simulink model "BaseEngineController_LS"  (Simulink 7.7)
settings: Solver=FixedStepDiscrete  StartTime=0.0  StopTime=10.0  RelTol=1e-3
PreLoadFcn:
  | try, eval([bdroot '_setup']); catch, eval('model_setup', ''); end
InitFcn:
  | try, eval([bdroot '_setup']); catch, eval('model_setup', ''); end
undefined symbols (not defined in the file): ECU555, High, motohawk_build_version, motohawk_trunc_name, motohawk_vardec_config_group, motohawk_vardec_path, True
libraries: MotoHawk_lib x1418, motohawk_control_primitives_lib x183, motohawk_engine_lib x32, simulink x21, motohawk_annotations_lib x9, AutoDoc_lib x8, simulink_extras x4, motohawk_ccp_examples_lib x1, motohawk_control_primitives_motoshare_lib x1
(part 11 of 27)

== system BaseEngineController_LS/Foreground/Control/ActuatorCharacterization/Electronic Throttle Controller/ETC Sticking Fault ==
  ETC Error : Inport
  ETC Setpoint Mode : Inport  Port=2
  Abs : Abs
  Logical Operator : Logic  AllPortsSameDT=off  OutDataTypeStr=boolean
  Relational Operator4 : RelationalOperator  Operator=>  ZeroCross=off  InputSameDT=on
  ShutDownAdaptMode1 : motohawk_control_primitives_lib/CompareTo  SystemSampleTime=-1  op===  val=0
  motohawk_calibration1 : MotoHawk_lib/Calibration & Probing Blocks/motohawk_calibration  nam='ETC_StickingThresh'  val=20  storage=Calibration  show_more=on  name_source=Use Parameter  data_type=double  read_level=1  write_level=1  ovr_cals=on  view_as=Number  enum_struct={'Disabled', 'Enabled'}  vector_style=Wide Row  use_help_units=on  help='Defines error limit between TPS_Request and TPS where ETC sticking fault will be set.'  units='%'  use_header_enum=off  row_header_enum={}  col_header_enum={}  use_min_max=on  min_val=-inf  max_val=inf  use_precision=off  precision=''  gain=1  offset=0  exp=1  use_mototune_group=on  mototune_group=motohawk_vardec_path(gcb)
  motohawk_fault_def1 : MotoHawk_lib/Fault Management Blocks/motohawk_fault_def  nam='ETC_Sticking'  mode=Sticky  id=[]  x=254  y=255  input_suspected=on  indeterminate=off  increment_xy=on  downsample_count=1  ovr_cals=on  ovr_actions=on  show_actions=off  action1_name=''  action1_cond=(None)  action2_name=''  action2_cond=(None)  action3_name=''  action3_cond=(None)  action4_name=''  action4_cond=(None)
  wires:
  Abs/1 -> Relational Operator4/1
  motohawk_calibration1/1 -> Relational Operator4/2
  ETC Error/1 -> Abs/1
  Logical Operator/1 -> motohawk_fault_def1/1
  Relational Operator4/1 -> Logical Operator/1
  ShutDownAdaptMode1/1 -> Logical Operator/2
  ETC Setpoint Mode/1 -> ShutDownAdaptMode1/1

== system BaseEngineController_LS/Foreground/Control/ActuatorCharacterization/Electronic Throttle Controller/ETCStallShutDown ==
  Constant1 : Constant  Value=150  OutDataTypeStr=Inherit: Inherit via back propagation  SampleTime=-1
  Logical Operator : Logic  AllPortsSameDT=off  OutDataTypeStr=boolean
  Relational Operator : RelationalOperator  Operator=>  ZeroCross=off  InputSameDT=on
  Relational Operator6 : RelationalOperator  Operator=>  OutDataTypeStr=boolean
  motohawk_ain_read : MotoHawk_lib/Analog I//O Blocks/motohawk_ain_read  nam='ECUP'  typ=uint16
  motohawk_calibration4 : MotoHawk_lib/Calibration & Probing Blocks/motohawk_calibration  nam='ETCShutdownTimerThresh'  val=5  storage=Calibration  show_more=on  name_source=Use Parameter  data_type=double  read_level=1  write_level=1  ovr_cals=on  view_as=Number  enum_struct={'Disabled', 'Enabled'}  vector_style=Wide Row  use_help_units=on  help='Time limit in Stall State after which ETC will shutdown.'  units='s'  use_header_enum=off  row_header_enum={}  col_header_enum={}  use_min_max=on  min_val=-inf  max_val=inf  use_precision=off  precision=''  gain=1  offset=0  exp=1  use_mototune_group=on  mototune_group=motohawk_vardec_path(gcb)
  motohawk_data_read : MotoHawk_lib/Data Storage Blocks/motohawk_data_read  source=Lookup By Name  structure=Scalar  operation=Read scalar from location by index  sz_vec=4  sz_row=2  sz_col=3  typ=double  nam='TimeSinceStall'  checkNull=on  struct_inst_name='Struct1'  struct_nam='MyStruct'
  motohawk_probe : MotoHawk_lib/Calibration & Probing Blocks/motohawk_probe  nam='ETCStallStateShutdown'  show_more=on  name_source=Use Parameter  read_level=1  view_as=Enumeration  enum_struct={'Disabled', 'Enabled'}  vector_style=Wide Row  use_help_units=off  help=''  units=''  use_header_enum=off  row_header_enum={}  col_header_enum={}  use_precision=off  precision=''  gain=1  offset=0  exp=1  use_mototune_group=on  mototune_group=motohawk_vardec_path(gcb)
  State : Outport
  wires:
  motohawk_data_read/1 -> Relational Operator6/1
  motohawk_calibration4/1 -> Relational Operator6/2
  motohawk_ain_read/1 -> Relational Operator/1
  Constant1/1 -> Relational Operator/2
  Relational Operator6/1 -> Logical Operator/1
  Relational Operator/1 -> Logical Operator/2
  Logical Operator/1 -> State/1, motohawk_probe/1

== system BaseEngineController_LS/Foreground/Control/ActuatorCharacterization/Electronic Throttle Controller/PID With Damper Terms (Tunable) ==
  Actual : Inport
  SetPoint : Inport  Port=2
  ResetITerm : Inport  Port=3
  Add : Sum  Inputs=+-
  DamperSwitch : Subsystem
  Ground2 : Ground
  IGain : Subsystem
  PGain : Subsystem
  PID With Damper Terms : Subsystem  Description=|  AncestorBlock=motohawk_control_primitives_lib/PID With Damper Terms  mask(PID with Damper Terms){samp_time=-1}
      | /* Name: ErrorGain Unit:mult ClassID:VAR StorageID:FLASH Access:RW4+RW3+NA2+NA1 TypeID:UINT4                   
      |    Gain:0.000000001 Min:0.000000000 Max:4.000000000 Format:10.9 UpdateID:REMOTE Help:"This gain is applied to "
      |    "the error term before it is used to calculate the P, I and D terms." VardecSig:6C */                       
      |                                                                                                                
      | /* Name: ITermLowerLim Unit:0 ClassID:VAR StorageID:FLASH Access:RW4+RW3+NA2+NA1 TypeID:SINT2 Gain:0.1         
      |    Min:-3276.8 Max:3276.7 Format:5.1 UpdateID:REMOTE Help:"Lower limit on the I-term value." VardecSig:6C */   
      |                                                                                                                
      | /* Name: ITermUpperLim ClassID:VAR StorageID:FLASH Access:RW4+RW3+NA2+NA1 TypeID:SINT2 Gain:0.1 Min:-3276.8    
      |    Max:3276.7 Format:5.1 UpdateID:REMOTE Help:"Upper limit on I-term value." VardecSig:6C */                   
      |                                                                                                                
      | /* Name: PIDOutLowerLim ClassID:VAR StorageID:FLASH Access:RW4+RW3+NA2+NA1 TypeID:SINT2 Gain:0.1               
      |    Min:-3276.8 Max:3276.7 Format:5.1 UpdateID:REMOTE Help:"Lower limit on PID output." VardecSig:6C */         
      |                                                                                                                
      | /* Name: PIDOutUpperLim ClassID:VAR StorageID:FLASH Access:RW4+RW3+NA2+NA1 TypeID:SINT2 Gain:0.1               
      |    Min:-3276.8 Max:3276.7 Format:3.1 UpdateID:REMOTE Help:"Upper limit on PID output." VardecSig:6C */         
      |                                                                                                                
      | /* Name: PIDError ClassID:VAR StorageID:RAM Access:RO4+RO3+NA2+NA1 TypeID:SINT2 Gain:1 Min:-32768.00           
      |    Max:32767.00 Format:4.2 UpdateID:BACKGND Help:"Current controller error input value." VardecSig:6C */       
      |                                                                                                                
      | /* Name: PTerm ClassID:VAR StorageID:RAM Access:RO4+RO3+NA2+NA1 TypeID:SINT2 Gain:1 Min:-32768.00              
      |    Max:32767.00 Format:4.2 UpdateID:BACKGND Help:"Current P-term value" VardecSig:6C */                        
      |                                                                                                                
      | /* Name: ITerm ClassID:VAR StorageID:RAM Access:RO4+RO3+NA2+NA1 TypeID:SINT2 Gain:1 Min:-32768.00              
      |    Max:32767.00 Format:4.2 UpdateID:BACKGND Help:"Current I-term value" VardecSig:6C */                        
      |                                                                                                                
      | /* Name: DTerm ClassID:VAR StorageID:RAM Access:RO4+RO3+NA2+NA1 TypeID:SINT2 Gain:1 Min:-32768.00              
      |    Max:32767.00 Format:4.2 UpdateID:BACKGND Help:"Current D-term value" VardecSig:6C */                        
      |                                                                                                                
      | /* Name: DamperTerm ClassID:VAR StorageID:RAM Access:RO4+RO3+NA2+NA1 TypeID:SINT2 Gain:1 Min:-32768.00         
      |    Max:32767.00 Format:4.2 UpdateID:BACKGND Help:"Current Damper-term value" VardecSig:6C */                   
      |                                                                                                                
      | /* Name: PIDOutput ClassID:VAR StorageID:FLASH Access:RW4+RW3+NA2+NA1 TypeID:SINT2 Gain:1 Min:-32768.00        
      |    Max:32767.00 Format:4.2 UpdateID:REMOTE Help:"PID current output." VardecSig:6C */
      mask prompts: samp_time "Sample Time"
      mask help:
      | Resettable PID controller with damper terms and limits on the I-term.
      |
      | If 'Sample Time' is -1, then extra code and RAM will be generated to dynamically calculate dt.
      mask Display:
      | patch([0 0 1 1], 0.5*[0 0.075 0.075 0], [230/255 0/255 0/255])
      | patch([0 0 1 1], 0.5*[0.025 0.05 0.05 0.025], [150/255 0/255 0/255])
      | patch([0 0 1 1], 0.5*[0 0.025 0.025 0], [0/255 0/255 0/255])
      | 
      | disp('\fontsize{16}\bf\itPIDD', 'texmode', 'on')
  Saturation (Tunable) : motohawk_control_primitives_lib/Saturation (Tunable)  SystemSampleTime=-1  prefix=prefix  units=units  grp=[grp ' | ' prefix ' PID Config']
  Sum : Sum  Inputs=++|  InputSameDT=on
  motohawk_calibration1 : MotoHawk_lib/Calibration & Probing Blocks/motohawk_calibration  nam=[prefix 'DGain']  val=.1  storage=Calibration  show_more=on  name_source=Use Parameter  data_type=Inherit from 'Default Value'  read_level=1  write_level=1  ovr_cals=on  view_as=Number  enum_struct={'Disabled', 'Enabled'}  vector_style=Wide Row  use_help_units=on  help='PID Derivative Gain'  units='mult'  use_header_enum=off  row_header_enum={}  col_header_enum={}  use_min_max=off  min_val=-inf  max_val=inf  use_precision=off  precision=''  gain=1  offset=0  exp=1  use_mototune_group=on  mototune_group=motohawk_vardec_path(gcb)
  motohawk_calibration3 : MotoHawk_lib/Calibration & Probing Blocks/motohawk_calibration  nam=[prefix 'IMin']  val=-50  storage=Calibration  show_more=on  name_source=Use Parameter  data_type=Inherit from 'Default Value'  read_level=1  write_level=1  ovr_cals=on  view_as=Number  enum_struct={'Disabled', 'Enabled'}  vector_style=Wide Row  use_help_units=on  help='PID Integrator Lower Limit'  units=units  use_header_enum=off  row_header_enum={}  col_header_enum={}  use_min_max=off  min_val=-inf  max_val=inf  use_precision=off  precision=''  gain=1  offset=0  exp=1  use_mototune_group=on  mototune_group=motohawk_vardec_path(gcb)
  motohawk_calibration4 : MotoHawk_lib/Calibration & Probing Blocks/motohawk_calibration  nam=[prefix 'IMax']  val=50  storage=Calibration  show_more=on  name_source=Use Parameter  data_type=Inherit from 'Default Value'  read_level=1  write_level=1  ovr_cals=on  view_as=Number  enum_struct={'Disabled', 'Enabled'}  vector_style=Wide Row  use_help_units=on  help='PID Integrator Upper Limit'  units=units  use_header_enum=off  row_header_enum={}  col_header_enum={}  use_min_max=off  min_val=-inf  max_val=inf  use_precision=off  precision=''  gain=1  offset=0  exp=1  use_mototune_group=on  mototune_group=motohawk_vardec_path(gcb)
  motohawk_calibration6 : MotoHawk_lib/Calibration & Probing Blocks/motohawk_calibration  nam=[prefix 'ErrorGain']  val=.5  storage=Calibration  show_more=on  name_source=Use Parameter  data_type=Inherit from 'Default Value'  read_level=1  write_level=1  ovr_cals=on  view_as=Number  enum_struct={'Disabled', 'Enabled'}  vector_style=Wide Row  use_help_units=on  help='PID Error Gain'  units='mult'  use_header_enum=off  row_header_enum={}  col_header_enum={}  use_min_max=off  min_val=-inf  max_val=inf  use_precision=off  precision=''  gain=1  offset=0  exp=1  use_mototune_group=on  mototune_group=motohawk_vardec_path(gcb)
  motohawk_calibration7 : MotoHawk_lib/Calibration & Probing Blocks/motohawk_calibration  nam=[prefix 'DampGainUp']  val=.01  storage=Calibration  show_more=on  name_source=Use Parameter  data_type=Inherit from 'Default Value'  read_level=1  write_level=1  ovr_cals=on  view_as=Number  enum_struct={'Disabled', 'Enabled'}  vector_style=Wide Row  use_help_units=on  help='PID Damper Gain - Up Direction'  units='mult'  use_header_enum=off  row_header_enum={}  col_header_enum={}  use_min_max=off  min_val=-inf  max_val=inf  use_precision=off  precision=''  gain=1  offset=0  exp=1  use_mototune_group=on  mototune_group=motohawk_vardec_path(gcb)
  motohawk_calibration8 : MotoHawk_lib/Calibration & Probing Blocks/motohawk_calibration  nam=[prefix 'DampGainDown']  val=.01  storage=Calibration  show_more=on  name_source=Use Parameter  data_type=Inherit from 'Default Value'  read_level=1  write_level=1  ovr_cals=on  view_as=Number  enum_struct={'Disabled', 'Enabled'}  vector_style=Wide Row  use_help_units=on  help='PID Damper Gain - Down Direction'  units='mult'  use_header_enum=off  row_header_enum={}  col_header_enum={}  use_min_max=off  min_val=-inf  max_val=inf  use_precision=off  precision=''  gain=1  offset=0  exp=1  use_mototune_group=on  mototune_group=motohawk_vardec_path(gcb)
  motohawk_interpolation_1d : MotoHawk_lib/Lookup Tables/motohawk_interpolation_1d  nam=[prefix 'DCOffset']  table_data=zeros(1,20)  show_more=on  data_type=Inherit from 'Table Data'  storage=NonAdaptive  read_level=1  write_level=1  ovr_cals=on  use_help=on  help='Duty cycle offset based on desired ETC position.'  units='%'  use_min_max=off  min_val=-inf  max_val=inf  use_precision=off  precision=''  gain=1  offset=0  exp=1  use_links=off  prelookup_block=''  output_name=''  use_mototune_group=on  mototune_group=motohawk_vardec_path(gcb)
  motohawk_prelookup : MotoHawk_lib/Lookup Tables/motohawk_prelookup  nam='ETC_Error'  breakpoint_data=[1:10]  show_more=on  data_type=Inherit from 'Table Data'  storage=Constant  read_level=1  write_level=1  ovr_cals=on  use_help=off  help=''  units=''  use_min_max=off  min_val=-inf  max_val=inf  use_precision=off  precision=''  gain=1  offset=0  exp=1  use_links=off  input_name=''  use_mototune_group=on  mototune_group=motohawk_vardec_path(gcb)
  motohawk_prelookup2 : MotoHawk_lib/Lookup Tables/motohawk_prelookup  nam='ETC_Setpoint'  breakpoint_data=[1:20]  show_more=on  data_type=Inherit from 'Table Data'  storage=Constant  read_level=1  write_level=1  ovr_cals=on  use_help=off  help=''  units=''  use_min_max=off  min_val=-inf  max_val=inf  use_precision=off  precision=''  gain=1  offset=0  exp=1  use_links=off  input_name=''  use_mototune_group=on  mototune_group=motohawk_vardec_path(gcb)
  motohawk_probe : MotoHawk_lib/Calibration & Probing Blocks/motohawk_probe  nam=[prefix 'Out']  show_more=on  name_source=Use Parameter  read_level=1  view_as=Number  enum_struct={'Disabled', 'Enabled'}  vector_style=Wide Row  use_help_units=on  help='PID Final Output'  units=units  use_header_enum=off  row_header_enum={}  col_header_enum={}  use_precision=off  precision=''  gain=1  offset=0  exp=1  use_mototune_group=on  mototune_group=motohawk_vardec_path(gcb)
  motohawk_probe1 : MotoHawk_lib/Calibration & Probing Blocks/motohawk_probe  nam=[prefix 'PTerm']  show_more=on  name_source=Use Parameter  read_level=1  view_as=Number  enum_struct={'Disabled', 'Enabled'}  vector_style=Wide Row  use_help_units=on  help='PID Proportional Term'  units=units  use_header_enum=off  row_header_enum={}  col_header_enum={}  use_precision=off  precision=''  gain=1  offset=0  exp=1  use_mototune_group=on  mototune_group=motohawk_vardec_path(gcb)
  motohawk_probe2 : MotoHawk_lib/Calibration & Probing Blocks/motohawk_probe  nam=[prefix 'ITerm']  show_more=on  name_source=Use Parameter  read_level=1  view_as=Number  enum_struct={'Disabled', 'Enabled'}  vector_style=Wide Row  use_help_units=on  help='PID Integrator Term'  units=units  use_header_enum=off  row_header_enum={}  col_header_enum={}  use_precision=off  precision=''  gain=1  offset=0  exp=1  use_mototune_group=on  mototune_group=motohawk_vardec_path(gcb)
  motohawk_probe3 : MotoHawk_lib/Calibration & Probing Blocks/motohawk_probe  nam=[prefix 'DTerm']  show_more=on  name_source=Use Parameter  read_level=1  view_as=Number  enum_struct={'Disabled', 'Enabled'}  vector_style=Wide Row  use_help_units=on  help='PID Derivative Term'  units=units  use_header_enum=off  row_header_enum={}  col_header_enum={}  use_precision=off  precision=''  gain=1  offset=0  exp=1  use_mototune_group=on  mototune_group=motohawk_vardec_path(gcb)
  motohawk_probe4 : MotoHawk_lib/Calibration & Probing Blocks/motohawk_probe  nam=[prefix 'Error']  show_more=on  name_source=Use Parameter  read_level=1  view_as=Number  enum_struct={'Disabled', 'Enabled'}  vector_style=Wide Row  use_help_units=on  help='PID Error Term'  units=units  use_header_enum=off  row_header_enum={}  col_header_enum={}  use_precision=off  precision=''  gain=1  offset=0  exp=1  use_mototune_group=on  mototune_group=motohawk_vardec_path(gcb)
  motohawk_probe5 : MotoHawk_lib/Calibration & Probing Blocks/motohawk_probe  nam=[prefix 'DampTerm']  show_more=on  name_source=Use Parameter  read_level=1  view_as=Number  enum_struct={'Disabled', 'Enabled'}  vector_style=Wide Row  use_help_units=on  help='PID Damper Term'  units=units  use_header_enum=off  row_header_enum={}  col_header_enum={}  use_precision=off  precision=''  gain=1  offset=0  exp=1  use_mototune_group=on  mototune_group=motohawk_vardec_path(gcb)
  motohawk_probe6 : MotoHawk_lib/Calibration & Probing Blocks/motohawk_probe  nam='ETC_Setpoint'  show_more=on  name_source=Use Parameter  read_level=1  view_as=Number  enum_struct={'Disabled', 'Enabled'}  vector_style=Wide Row  use_help_units=on  help='Commanded electronic throttle position'  units='%'  use_header_enum=off  row_header_enum={}  col_header_enum={}  use_precision=off  precision=''  gain=1  offset=0  exp=1  use_mototune_group=on  mototune_group=motohawk_vardec_path(gcb)
  Out : Outport
  wires:
  Saturation (Tunable)/1 -> motohawk_probe/1, Out/1
  PID With Damper Terms/6(Dmp_term) -> motohawk_probe5/1
  motohawk_calibration8/1 -> PID With Damper Terms/8(k_Dmp,d)
  motohawk_calibration7/1 -> PID With Damper Terms/7(k_Dmp,u)
  PID With Damper Terms/2(Err) -> motohawk_probe4/1
  PID With Damper Terms/5(D_term) -> motohawk_probe3/1
  PID With Damper Terms/4(I_term) -> motohawk_probe2/1
  motohawk_calibration4/1 -> PID With Damper Terms/11(I_max)
  motohawk_calibration3/1 -> PID With Damper Terms/10(I_min)
  motohawk_calibration6/1 -> PID With Damper Terms/3(k_Err)
  PID With Damper Terms/1(Out) -> Sum/2
  SetPoint/1 -> motohawk_prelookup2/1, Add/1, PID With Damper Terms/2(SetPt), motohawk_probe6/1
  Actual/1 -> PID With Damper Terms/1(Actual), Add/2, DamperSwitch/1(TPS)
  PID With Damper Terms/3(P_term) -> motohawk_probe1/1
  PGain/1(PGain) -> PID With Damper Terms/4(k_P)
  IGain/1(IGain) -> PID With Damper Terms/5(k_I)
  motohawk_calibration1/1 -> PID With Damper Terms/6(k_D)
  Ground2/1 -> PID With Damper Terms/9(IC)
  ResetITerm/1 -> PID With Damper Terms/12(I_reset)
  Sum/1 -> Saturation (Tunable)/1
  motohawk_interpolation_1d/1 -> Sum/1
  motohawk_prelookup/1 -> PGain/1(ErrorIdx), IGain/1(ErrorIdx)
  Add/1 -> motohawk_prelookup/1
  motohawk_prelookup2/1 -> motohawk_interpolation_1d/1
  DamperSwitch/1(SwitchState) -> PID With Damper Terms/13(DamperSwitchState)

== system BaseEngineController_LS/Foreground/Control/ActuatorCharacterization/Electronic Throttle Controller/Reset TasksComplete To True ==
  Trigger : TriggerPort
  Constant2 : Constant  Value=true  SampleTime=-1
  motohawk_data_write : MotoHawk_lib/Data Storage Blocks/motohawk_data_write  source=Lookup By Name  structure=Scalar  operation=Write entire data structure at once  sz_vec=-1  sz_row=3  sz_col=2  typ=boolean  nam='ShutDownTasksComplete'  checkNull=off  write_read_only=off  struct_inst_name='Struct1'  struct_name='MyStruct'
  wires:
  Constant2/1 -> motohawk_data_write/1

== system BaseEngineController_LS/Foreground/Control/ActuatorCharacterization/Electronic Throttle Controller/Setpoint Manager ==
  TPS Position : Inport
  Controller Setpoint : Inport  Port=2
  Setpoint Mode : Inport  Port=3
  Add : Sum  Inputs=-+
  Add1 : Sum
  Add2 : Sum
  Constant1 : Constant  Value=10  SampleTime=-1
  Constant2 : Constant  Value=-5  SampleTime=-1
  Constant7 : Constant  Value=100  SampleTime=-1
  Multiport Switch : MultiPortSwitch  DataPortOrder=Zero-based contiguous  zeroidx=on
  PassThrough : Subsystem  TreatAsAtomicUnit=on
  ShutDownAdaptMode1 : motohawk_control_primitives_lib/CompareTo  SystemSampleTime=-1  op===  val=1
  Tuning : Subsystem
  Variable Rate Limiter : Subsystem  mask(Variable Rate Limiter){}
      mask help: Variable Rate Limiter Block
      mask Display:
      | patch([0 0 1 1], [0 0.075 0.075 0], [230/255 0/255 0/255])
      | patch([0 0 1 1], [0.025 0.05 0.05 0.025], [150/255 0/255 0/255])
      | patch([0 0 1 1], [0 0.025 0.025 0], [0/255 0/255 0/255])
      | 
      | disp(['RATE \nLIMITER']);
  motohawk_calibration2 : MotoHawk_lib/Calibration & Probing Blocks/motohawk_calibration  nam='ETC_LoAdaptRateLimit'  val=-40  storage=Calibration  show_more=on  name_source=Use Parameter  data_type=double  read_level=1  write_level=1  ovr_cals=on  view_as=Number  enum_struct={'Disabled', 'Enabled'}  vector_style=Wide Row  use_help_units=on  help='Dictates the rate at which the ETC setpoint is decreased during shutdown to perform a low TPS adapt.'  units='%/s'  use_header_enum=off  row_header_enum={}  col_header_enum={}  use_min_max=on  min_val=-inf  max_val=inf  use_precision=off  precision=''  gain=1  offset=0  exp=1  use_mototune_group=on  mototune_group=motohawk_vardec_path(gcb)
  motohawk_data_read1 : MotoHawk_lib/Data Storage Blocks/motohawk_data_read  source=Lookup By Name  structure=Scalar  operation=Read scalar from location by index  sz_vec=4  sz_row=2  sz_col=3  typ=double  nam='ETC_SpringTestHiThresh'  checkNull=on  struct_inst_name='Struct1'  struct_nam='MyStruct'
  motohawk_data_read3 : MotoHawk_lib/Data Storage Blocks/motohawk_data_read  source=Lookup By Name  structure=Scalar  operation=Read scalar from location by index  sz_vec=4  sz_row=2  sz_col=3  typ=double  nam='ETC_ShutdownLoAdaptError'  checkNull=on  struct_inst_name='Struct1'  struct_nam='MyStruct'
  ETC_Setpoint : Outport
  ETC_Error : Outport  Port=2
  wires:
  Tuning/1(SetpointOut) -> Multiport Switch/2
  Add1/1 -> Multiport Switch/4
  Variable Rate Limiter/1(output) -> Multiport Switch/3
  PassThrough/1(Out1) -> Variable Rate Limiter/1(input)
  Add2/1 -> PassThrough/1(In1)
  Constant7/1 -> Variable Rate Limiter/2(rise rate)
  motohawk_calibration2/1 -> Variable Rate Limiter/3(fall rate)
  Controller Setpoint/1 -> Tuning/1(Setpoint)
  Setpoint Mode/1 -> Multiport Switch/1, ShutDownAdaptMode1/1
  ShutDownAdaptMode1/1 -> PassThrough/Enable
  Add/1 -> ETC_Error/1
  Multiport Switch/1 -> ETC_Setpoint/1, Add/2
  TPS Position/1 -> Add/1
  motohawk_data_read1/1 -> Add1/2
  Constant1/1 -> Add1/1
  motohawk_data_read3/1 -> Add2/2
  Constant2/1 -> Add2/1

== system BaseEngineController_LS/Foreground/Control/ActuatorCharacterization/Electronic Throttle Controller/State  Manager ==
  Constant1 : Constant  Value=150  OutDataTypeStr=Inherit: Inherit via back propagation  SampleTime=-1
  Logical Operator2 : Logic  Operator=NOT  AllPortsSameDT=off  OutDataTypeStr=boolean
  Logical Operator3 : Logic  Inputs=3  AllPortsSameDT=off  OutDataTypeStr=boolean
  Relational Operator : RelationalOperator  Operator=<  ZeroCross=off  InputSameDT=on
  Reset TasksComplete To False : Subsystem  TreatAsAtomicUnit=on
  Stall : motohawk_control_primitives_lib/CompareTo  SystemSampleTime=-1  op===  val=1
  Time Since Enabled (With Input)1 : motohawk_control_primitives_lib/Time Since Enabled (With Input)1  SystemSampleTime=-1  nam='ETCShutDownTimer'  samp_time=-1  init=0  upperlim=16000
  motohawk_ain_read : MotoHawk_lib/Analog I//O Blocks/motohawk_ain_read  nam='ECUP'  typ=uint16
  motohawk_data_read1 : MotoHawk_lib/Data Storage Blocks/motohawk_data_read  source=Lookup By Name  structure=Scalar  operation=Read entire data structure at once  sz_vec=4  sz_row=2  sz_col=3  typ=boolean  nam='MPRD'  checkNull=on  struct_inst_name='Struct1'  struct_nam='MyStruct'
  motohawk_data_read2 : MotoHawk_lib/Data Storage Blocks/motohawk_data_read  source=Lookup By Name  structure=Scalar  operation=Read entire data structure at once  sz_vec=4  sz_row=2  sz_col=3  typ=boolean  nam='ShutDownTasksComplete'  checkNull=on  struct_inst_name='Struct1'  struct_nam='MyStruct'
  motohawk_data_read3 : MotoHawk_lib/Data Storage Blocks/motohawk_data_read  source=Lookup By Name  structure=Scalar  operation=Read entire data structure at once  sz_vec=4  sz_row=2  sz_col=3  typ=uint8  nam='EngineState'  checkNull=on  struct_inst_name='Struct1'  struct_nam='MyStruct'
  motohawk_probe1 : MotoHawk_lib/Calibration & Probing Blocks/motohawk_probe  nam='ETC_ShutDownTimer'  show_more=on  name_source=Use Parameter  read_level=1  view_as=Number  enum_struct={'Disabled', 'Enabled'}  vector_style=Wide Row  use_help_units=off  help=''  units=''  use_header_enum=off  row_header_enum={}  col_header_enum={}  use_precision=off  precision=''  gain=1  offset=0  exp=1  use_mototune_group=on  mototune_group=motohawk_vardec_path(gcb)
  motohawk_probe2 : MotoHawk_lib/Calibration & Probing Blocks/motohawk_probe  nam='ETC_ECUPState'  show_more=on  name_source=Use Parameter  read_level=1  view_as=Number  enum_struct={'Disabled', 'Enabled'}  vector_style=Wide Row  use_help_units=off  help=''  units=''  use_header_enum=off  row_header_enum={}  col_header_enum={}  use_precision=off  precision=''  gain=1  offset=0  exp=1  use_mototune_group=on  mototune_group=motohawk_vardec_path(gcb)
  ECUP State : Outport
  ECUP Timer : Outport  Port=2
  wires:
  Relational Operator/1 -> Time Since Enabled (With Input)1/1, Logical Operator3/3
  motohawk_ain_read/1 -> Relational Operator/1
  Constant1/1 -> Relational Operator/2
  motohawk_data_read2/1 -> Logical Operator2/1
  Logical Operator2/1 -> Logical Operator3/2
  motohawk_data_read3/1 -> Stall/1
  Stall/1 -> Logical Operator3/1
  Logical Operator3/1 -> ECUP State/1, motohawk_probe2/1
  Time Since Enabled (With Input)1/1 -> ECUP Timer/1, motohawk_probe1/1
  motohawk_data_read1/1 -> Reset TasksComplete To False/Trigger

== system BaseEngineController_LS/Foreground/Control/ActuatorCharacterization/Injector Characterization/DeltaPressureIndex ==
  Inputs : Inport
  const ref to atm : Fcn  Expr=u(1) + u(2) - u(3)
  motohawk_prelookup1 : MotoHawk_lib/Lookup Tables/motohawk_prelookup  nam='InjDeltaPress09'  breakpoint_data=[300 315 325 350 365 385 415 430 450]  show_more=on  data_type=Inherit from 'Table Data'  storage=Constant  read_level=1  write_level=1  ovr_cals=on  use_help=on  help=''  units=''  use_min_max=off  min_val=-inf  max_val=inf  use_precision=on  precision=''  gain=1  offset=0  exp=1  use_links=off  input_name=''  use_mototune_group=on  mototune_group=motohawk_vardec_path(gcb)
  motohawk_probe2 : MotoHawk_lib/Calibration & Probing Blocks/motohawk_probe  nam='FuelDeltaPress'  show_more=on  name_source=Use Parameter  read_level=1  view_as=Number  enum_struct={'Disabled', 'Enabled'}  vector_style=Wide Row  use_help_units=on  help='Fuel Delta Pressure - across the fuel injector'  units='kPa'  use_header_enum=off  row_header_enum={}  col_header_enum={}  use_precision=off  precision=''  gain=1  offset=0  exp=1  use_mototune_group=on  mototune_group=motohawk_vardec_path(gcb)
  Index : Outport
  wires:
  const ref to atm/1 -> motohawk_probe2/1, motohawk_prelookup1/1
  Inputs/1 -> const ref to atm/1
  motohawk_prelookup1/1 -> Index/1

== system BaseEngineController_LS/Foreground/Control/ActuatorCharacterization/SequenceCutPattern/Hard Cycle Cut Pattern ==
  Cycle1CutPatter : Subsystem
  Cycle2CutPatter : Subsystem
  Cycle3CutPatter : Subsystem
  Cycle4CutPatter : Subsystem
  Mux1 : Mux
  Pattern : Outport
  wires:
  Cycle4CutPatter/1(Out) -> Mux1/4
  Cycle3CutPatter/1(Out) -> Mux1/3
  Cycle2CutPatter/1(Out) -> Mux1/2
  Cycle1CutPatter/1(Out) -> Mux1/1
  Mux1/1 -> Pattern/1

== system BaseEngineController_LS/Foreground/Control/ActuatorCharacterization/SequenceCutPattern/Medium Cycle Cut Pattern ==
  Cycle1CutPatter : Subsystem
  Cycle2CutPatter : Subsystem
  Cycle3CutPatter : Subsystem
  Cycle4CutPatter : Subsystem
  Mux1 : Mux
  Pattern : Outport
  wires:
  Mux1/1 -> Pattern/1
  Cycle1CutPatter/1(Out) -> Mux1/1
  Cycle2CutPatter/1(Out) -> Mux1/2
  Cycle3CutPatter/1(Out) -> Mux1/3
  Cycle4CutPatter/1(Out) -> Mux1/4

== system BaseEngineController_LS/Foreground/Control/ActuatorCharacterization/SequenceCutPattern/PassThrough1 ==
  In1 : Inport
  Enable : EnablePort  StatesWhenEnabling=reset
  Out1 : Outport  OutputWhenDisabled=reset  InitialOutput=[0]
  wires:
  In1/1 -> Out1/1

== system BaseEngineController_LS/Foreground/Control/ActuatorCharacterization/SequenceCutPattern/PassThrough2 ==
  In1 : Inport
  Enable : EnablePort
  Out1 : Outport  InitialOutput=[0]
  wires:
  In1/1 -> Out1/1

== system BaseEngineController_LS/Foreground/Control/ActuatorCharacterization/SequenceCutPattern/PassThrough3 ==
  In1 : Inport
  Enable : EnablePort
  Out1 : Outport  OutputWhenDisabled=reset  InitialOutput=[0]
  wires:
  In1/1 -> Out1/1

== system BaseEngineController_LS/Foreground/Control/ActuatorCharacterization/SequenceCutPattern/PassThrough4 ==
  In1 : Inport
  Enable : EnablePort  StatesWhenEnabling=reset
  Data Type Conversion : DataTypeConversion  SaturateOnIntegerOverflow=on  RndMeth=Zero
  Out1 : Outport  OutputWhenDisabled=reset  InitialOutput=[0]
  wires:
  In1/1 -> Data Type Conversion/1
  Data Type Conversion/1 -> Out1/1

== system BaseEngineController_LS/Foreground/Control/ActuatorCharacterization/SequenceCutPattern/PassThrough5 ==
  In1 : Inport
  Enable : EnablePort  StatesWhenEnabling=reset
  Data Type Conversion1 : DataTypeConversion  SaturateOnIntegerOverflow=on  RndMeth=Zero
  Out1 : Outport  OutputWhenDisabled=reset  InitialOutput=[0]
  wires:
  In1/1 -> Data Type Conversion1/1
  Data Type Conversion1/1 -> Out1/1

== system BaseEngineController_LS/Foreground/Control/ActuatorCharacterization/SequenceCutPattern/SequenceCutMachine ==
  Cycles : Inport
  Enable : EnablePort  StatesWhenEnabling=reset
  Demux : Demux
  Multiport Switch : MultiPortSwitch  Inputs=4  zeroidx=off  SaturateOnIntegerOverflow=on
  SequencyCutMachine : Subsystem  TreatAsAtomicUnit=on
  Unit Delay1 : UnitDelay  X0=1  SampleTime=-1
  Unit Delay2 : UnitDelay  X0=1  SampleTime=-1
  motohawk_trigger : MotoHawk_lib/Trigger Blocks/motohawk_trigger  Tag=Trigger  trigger=FGND_TDC1_EVENT  function_name=Trigger_FGND_TDC1_EVENT_10311p001  priority_order=0  inherited=on  run_disabled=off  override_app_monitor=off  target=ECU555_80
  Out1 : Outport  InitialOutput=0
  wires:
  SequencyCutMachine/1(CylsToCut) -> Out1/1
  Unit Delay1/1 -> SequencyCutMachine/2(CurrentCount)
  SequencyCutMachine/2(CycleCounter) -> Unit Delay1/1
  Multiport Switch/1 -> SequencyCutMachine/1(CutArray)
  motohawk_trigger/1 -> SequencyCutMachine/Trigger
  Demux/1 -> Multiport Switch/2
  Demux/2 -> Multiport Switch/3
  Demux/3 -> Multiport Switch/4
  Demux/4 -> Multiport Switch/5
  Cycles/1 -> Demux/1
  SequencyCutMachine/3(CycleNumber) -> Unit Delay2/1
  Unit Delay2/1 -> SequencyCutMachine/3(CurrentCycle), Multiport Switch/1

== system BaseEngineController_LS/Foreground/Control/ActuatorCharacterization/SequenceCutPattern/Soft Cycle Cut Pattern ==
  Cycle1CutPatter : Subsystem
  Cycle2CutPatter : Subsystem
  Cycle3CutPatter : Subsystem
  Cycle4CutPatter : Subsystem
  Mux1 : Mux
  Pattern : Outport
  wires:
  Cycle4CutPatter/1(Out) -> Mux1/4
  Cycle3CutPatter/1(Out) -> Mux1/3
  Cycle2CutPatter/1(Out) -> Mux1/2
  Cycle1CutPatter/1(Out) -> Mux1/1
  Mux1/1 -> Pattern/1

== system BaseEngineController_LS/Foreground/Control/Controller/Crank/CrankFueling ==
  RPMIdx : Inport
  ECTIdx : Inport  Port=2
  APP : Inport  Port=3
  TPS : Inport  Port=4
  IATIdx : Inport  Port=5
  OXYIdx : Inport  Port=6
  Add : Sum
  ClearFloodFueling : Constant  Value=0  OutDataTypeStr=Inherit: Inherit via back propagation  SampleTime=-1
  ClearFloodFueling1 : Constant  OutDataTypeStr=Inherit: Inherit via back propagation  SampleTime=-1
  ClearFloodFueling3 : Constant  Value=0  OutDataTypeStr=Inherit: Inherit via back propagation  SampleTime=-1
  Gain : Gain  Gain=.01
  Multiport Switch1 : MultiPortSwitch  DataPortOrder=Zero-based contiguous  Inputs=2  zeroidx=on
  Multiport Switch2 : MultiPortSwitch  DataPortOrder=Zero-based contiguous  Inputs=2  zeroidx=on
  Product : Product  RndMeth=Zero
  Product1 : Product  RndMeth=Zero
  Product2 : Product  Inputs=3  RndMeth=Zero
  Relational Operator : RelationalOperator  InputSameDT=on
  Switch : Switch  Threshold=.5  SaturateOnIntegerOverflow=on
  motohawk_calibration1 : MotoHawk_lib/Calibration & Probing Blocks/motohawk_calibration  nam='OpenThrottleFPCScalar'  val=1  storage=Calibration  show_more=on  name_source=Use Parameter  data_type=Inherit from 'Default Value'  read_level=1  write_level=1  ovr_cals=on  view_as=Number  enum_struct={'Disabled', 'Enabled'}  vector_style=Wide Row  use_help_units=on  help="'Crank FPC is scaled up with throttle opening for mechanical throttle systems, this parameter sets the gain for this relationship.  CrankFPC=CrankFPC*(1+TPS/100*FPCScalar).'"  units='Mult'  use_header_enum=off  row_header_enum={}  col_header_enum={}  use_min_max=off  min_val=-inf  max_val=inf  use_precision=off  precision=''  gain=1  offset=0  exp=1  use_mototune_group=on  mototune_group=motohawk_vardec_path(gcb)
  motohawk_calibration2 : MotoHawk_lib/Calibration & Probing Blocks/motohawk_calibration  nam='ClearFloodThreshold'  val=80  storage=Calibration  show_more=on  name_source=Use Parameter  data_type=Inherit from 'Default Value'  read_level=1  write_level=1  ovr_cals=on  view_as=Number  enum_struct={'Disabled', 'Enabled'}  vector_style=Wide Row  use_help_units=on  help='In crank mode, throttle commands greater than this threshold will disable crank fueling.'  units='Mult'  use_header_enum=off  row_header_enum={}  col_header_enum={}  use_min_max=off  min_val=-inf  max_val=inf  use_precision=off  precision=''  gain=1  offset=0  exp=1  use_mototune_group=on  mototune_group=motohawk_vardec_path(gcb)
  motohawk_data_read1 : MotoHawk_lib/Data Storage Blocks/motohawk_data_read  source=Lookup By Name  structure=Scalar  operation=Read scalar from location by index  sz_vec=4  sz_row=2  sz_col=3  typ=boolean  nam='AirControlSource'  checkNull=on  struct_inst_name='Struct1'  struct_nam='MyStruct'
  motohawk_interpolation_1d : MotoHawk_lib/Lookup Tables/motohawk_interpolation_1d  nam='CrankFPC_IATMult'  table_data=[1 1 1 1 1]  show_more=on  data_type=Inherit from 'Table Data'  storage=NonAdaptive  read_level=1  write_level=1  ovr_cals=on  use_help=on  help='Crank fuel IAT ultiplier'  units=''  use_min_max=on  min_val=0  max_val=100  use_precision=on  precision=''  gain=1  offset=0  exp=1  use_links=off  prelookup_block=''  output_name=''  use_mototune_group=on  mototune_group=motohawk_vardec_path(gcb)
  motohawk_interpolation_1d1 : MotoHawk_lib/Lookup Tables/motohawk_interpolation_1d  nam='CrankFPC_OXYMult'  table_data=[1 1 1.2 1.3 1.4]  show_more=on  data_type=Inherit from 'Table Data'  storage=NonAdaptive  read_level=1  write_level=1  ovr_cals=on  use_help=on  help='Crank fuel oxygentation multiplier'  units=''  use_min_max=on  min_val=0  max_val=100  use_precision=on  precision=''  gain=1  offset=0  exp=1  use_links=off  prelookup_block=''  output_name=''  use_mototune_group=on  mototune_group=motohawk_vardec_path(gcb)
  motohawk_interpolation_2d : MotoHawk_lib/Lookup Tables/motohawk_interpolation_2d  nam='CrankFPC'  table_data=[320 200 120 110 50;300 180 129 110 50;250 160 120 100 60;200 130 120 80 60;150 140 130 90 60]  show_more=on  data_type=Inherit from 'Table Data'  storage=NonAdaptive  read_level=1  write_level=1  ovr_cals=on  use_help=on  help='Liquid fuel supplied during crank.'  units='mg/cyl'  use_min_max=on  min_val=0  max_val=inf  use_precision=on  precision=''  gain=1  offset=0  exp=1  use_links=off  row_prelookup_block=''  col_prelookup_block=''  output_name=''  use_mototune_group=on  mototune_group=motohawk_vardec_path(gcb)
  FPC : Outport
  wires:
  ClearFloodFueling/1 -> Switch/1
  Relational Operator/1 -> Switch/2
  motohawk_calibration2/1 -> Relational Operator/2
  ECTIdx/1 -> motohawk_interpolation_2d/1
  RPMIdx/1 -> motohawk_interpolation_2d/2
  Add/1 -> Product/1
  Product1/1 -> Add/2
  ClearFloodFueling1/1 -> Add/1
  Gain/1 -> Product1/2
  Product/1 -> FPC/1
  Switch/1 -> Product/2
  motohawk_data_read1/1 -> Multiport Switch1/1, Multiport Switch2/1
  Multiport Switch1/1 -> Relational Operator/1, Gain/1
  APP/1 -> Multiport Switch1/2
  TPS/1 -> Multiport Switch1/3
  Multiport Switch2/1 -> Product1/1
  motohawk_calibration1/1 -> Multiport Switch2/3
  ClearFloodFueling3/1 -> Multiport Switch2/2
  IATIdx/1 -> motohawk_interpolation_1d/1
  OXYIdx/1 -> motohawk_interpolation_1d1/1
  motohawk_interpolation_2d/1 -> Product2/1
  motohawk_interpolation_1d/1 -> Product2/2
  motohawk_interpolation_1d1/1 -> Product2/3
  Product2/1 -> Switch/3

== system BaseEngineController_LS/Foreground/Control/Controller/Crank/CrankIAC ==
  RPMIdx : Inport
  ECTIdx : Inport  Port=2
  IATIdx : Inport  Port=3
  OXYIdx : Inport  Port=4
  Product : Product  Inputs=3  RndMeth=Zero
  motohawk_interpolation_1d : MotoHawk_lib/Lookup Tables/motohawk_interpolation_1d  nam='CrankIAC_IATMult'  table_data=[1 1 1 1 1]  show_more=on  data_type=Inherit from 'Table Data'  storage=NonAdaptive  read_level=1  write_level=1  ovr_cals=on  use_help=off  help=''  units=''  use_min_max=on  min_val=0  max_val=100  use_precision=on  precision=''  gain=1  offset=0  exp=1  use_links=off  prelookup_block=''  output_name=''  use_mototune_group=on  mototune_group=motohawk_vardec_path(gcb)
  motohawk_interpolation_1d1 : MotoHawk_lib/Lookup Tables/motohawk_interpolation_1d  nam='CrankIAC_OXYMult'  table_data=[1 1 1 1 1]  show_more=on  data_type=Inherit from 'Table Data'  storage=NonAdaptive  read_level=1  write_level=1  ovr_cals=on  use_help=off  help=''  units=''  use_min_max=on  min_val=0  max_val=100  use_precision=on  precision=''  gain=1  offset=0  exp=1  use_links=off  prelookup_block=''  output_name=''  use_mototune_group=on  mototune_group=motohawk_vardec_path(gcb)
  motohawk_interpolation_2d : MotoHawk_lib/Lookup Tables/motohawk_interpolation_2d  nam='CrankIAC'  table_data=ones(5,5)  show_more=on  data_type=Inherit from 'Table Data'  storage=NonAdaptive  read_level=1  write_level=1  ovr_cals=on  use_help=on  help='Base IAC % While Cranking'  units='%'  use_min_max=on  min_val=0  max_val=100  use_precision=on  precision=''  gain=1  offset=0  exp=1  use_links=off  row_prelookup_block=''  col_prelookup_block=''  output_name=''  use_mototune_group=on  mototune_group=motohawk_vardec_path(gcb)
  IAC % : Outport
  wires:
  motohawk_interpolation_2d/1 -> Product/1
  motohawk_interpolation_1d/1 -> Product/2
  motohawk_interpolation_1d1/1 -> Product/3
  Product/1 -> IAC %/1
  ECTIdx/1 -> motohawk_interpolation_2d/1
  RPMIdx/1 -> motohawk_interpolation_2d/2
  IATIdx/1 -> motohawk_interpolation_1d/1
  OXYIdx/1 -> motohawk_interpolation_1d1/1

== system BaseEngineController_LS/Foreground/Control/Controller/Crank/IAC Characterization ==
  IAC % : Inport
  Constant : Constant  Value=0
  Constant1 : Constant  Value=100
  Sum : Sum  Inputs=|+-
  Switch : Switch  Criteria=u2 > Threshold
  Switch1 : Switch  Criteria=u2 > Threshold
  motohawk_data_read : MotoHawk_lib/Data Storage Blocks/motohawk_data_read  source=Lookup By Name  structure=Scalar  operation=Read scalar from location by index  sz_vec=4  sz_row=2  sz_col=3  typ=uint8  nam='IACType'  checkNull=on  struct_inst_name='MyData'  struct_nam='MyStruct'
  IAC-P : Outport
  IAC-S : Outport  Port=2
  wires:
  motohawk_data_read/1 -> Switch/2, Switch1/2
  Switch/1 -> IAC-P/1
  IAC %/1 -> Switch/3, Switch/1, Sum/2
  Switch1/1 -> IAC-S/1
  Constant/1 -> Switch1/3
  Constant1/1 -> Sum/1
  Sum/1 -> Switch1/1

== system BaseEngineController_LS/Foreground/Control/Controller/Merge/FuelPump ==
  FuelP : Inport
  Logical Operator : Logic  Operator=OR  AllPortsSameDT=off  OutDataTypeStr=boolean
  OFF : Constant  Value=0  OutDataTypeStr=boolean
  Switch : Switch  Threshold=1  ZeroCross=off  SaturateOnIntegerOverflow=on  InputSameDT=on
  motohawk_data_read : MotoHawk_lib/Data Storage Blocks/motohawk_data_read  source=Lookup By Name  structure=Scalar  operation=Read scalar from location by index  sz_vec=4  sz_row=2  sz_col=3  typ=boolean  nam='DelayedEngineShutdownAction'  checkNull=on  struct_inst_name='Struct1'  struct_nam='MyStruct'
  motohawk_data_read1 : MotoHawk_lib/Data Storage Blocks/motohawk_data_read  source=Lookup By Name  structure=Scalar  operation=Read scalar from location by index  sz_vec=4  sz_row=2  sz_col=3  typ=boolean  nam='EngineShutdownAction'  checkNull=on  struct_inst_name='Struct1'  struct_nam='MyStruct'
  Out : Outport
  wires:
  motohawk_data_read/1 -> Logical Operator/1
  motohawk_data_read1/1 -> Logical Operator/2
  OFF/1 -> Switch/1
  Switch/1 -> Out/1
  FuelP/1 -> Switch/3
  Logical Operator/1 -> Switch/2
